simulink model "RuleBasedTractionControl"  (R2019b)
settings: Solver=ode1  StartTime=0.0  StopTime=inf  FixedStep=0.0002  RelTol=1e-3
PreLoadFcn:
  | vehicle = 'Car'; if ~length(which('cmself')), cmenv; end
  | RuleBasedTractionControl_bus
InitFcn:
  | vehicle = 'Car'; if ~length(which('cmself')), cmenv; end
  | RuleBasedTractionControl_bus
model workspace (MAT data in the model file):
  SLIP_FRONT = [0 0.05 0.1 0.15 0.25 0.5 1 2 10]
  TORQUE_DELTA_FRONT = [0 0.03 0.07 0.09 0.15 0.25 0.5 0.8 1]
libraries: CarMaker4SL x4
(part 2 of 2)

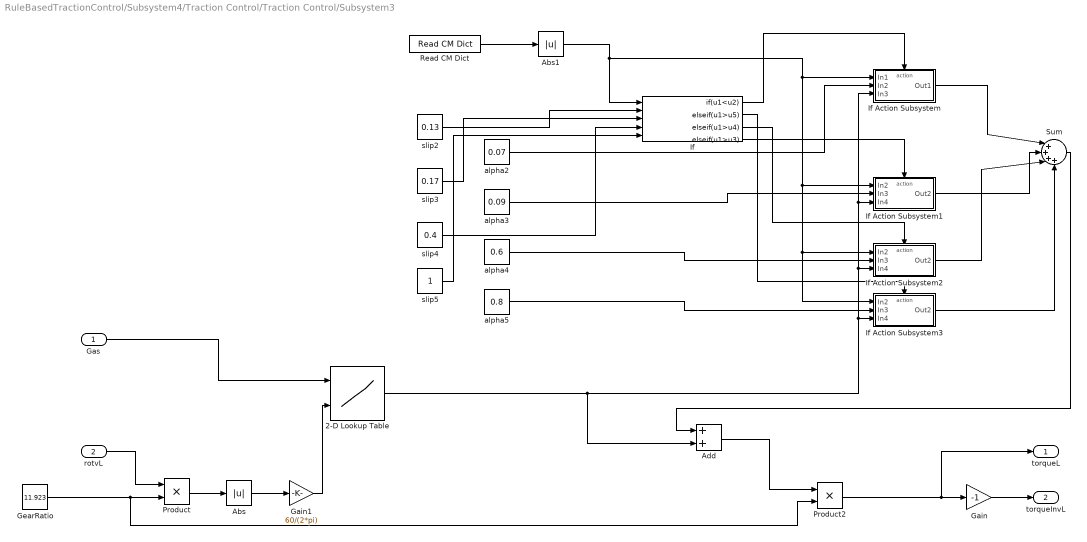
== system RuleBasedTractionControl/Subsystem4/Traction Control/Traction Control/Subsystem3 ==
  Gas : Inport
  rotvL : Inport  Port=2
  2-D Lookup Table : Lookup_n-D  BreakpointsForDimension1=[0 0.2 0.4 0.6 0.8 1]  BreakpointsForDimension2=[0 2000 4000 6000 8000 10000 12000 14000 15000 16000 17000 18000 20000 22000]  Table=[0 0 0 0 0 0 0 0 0 0 0 0 0 0;4 4 4 4 4 4 4 4 4 4 4 4 3 0;8 8 8 8 8 8 8 8 8 8 8 8 6 0;13 13 13 13 13 13 13 13 13 12 12 11 9 0;17 17 17 17 17 17 17 17 17 16 16 15 12 0;21 21 21 21 21 21 21 21 21 20 20 19 15 0]  InternalRulePriority=Speed  RndMeth=Simplest  InputSameDT=on
  Abs : Abs
  Abs1 : Abs
  Add : Sum
  Gain : Gain  Gain=-1
  Gain1 : Gain  Gain=60/(2*pi)
  GearRatio : Constant  Value=11.923
  If : If  NumInputs=5  IfExpression=u1<u2  ElseIfExpressions=u1>u5, u1>u4, u1>u3  ShowElse=off
  If Action Subsystem : Subsystem  TreatAsAtomicUnit=on
  If Action Subsystem1 : Subsystem  TreatAsAtomicUnit=on
  If Action Subsystem2 : Subsystem  TreatAsAtomicUnit=on
  If Action Subsystem3 : Subsystem  TreatAsAtomicUnit=on
  Product : Product
  Product2 : Product
  Read CM Dict : CarMaker4SL/Read CM Dict  xname=Car.LongSlipRR  xsync=off
  Sum : Sum  Inputs=|++++
  alpha2 : Constant  Value=0.07
  alpha3 : Constant  Value=0.09
  alpha4 : Constant  Value=0.6
  alpha5 : Constant  Value=0.8
  slip2 : Constant  Value=0.13
  slip3 : Constant  Value=0.17
  slip4 : Constant  Value=0.4
  slip5 : Constant
  torqueL : Outport
  torqueInvL : Outport  Port=2
  wires:
  Gain/1 -> torqueInvL/1
  Product/1 -> Abs/1
  Gas/1 -> 2-D Lookup Table/1
  GearRatio/1 -> Product2/2, Product/2
  rotvL/1 -> Product/1
  Product2/1 -> Gain/1, torqueL/1
  Abs/1 -> Gain1/1
  Gain1/1 -> 2-D Lookup Table/2
  2-D Lookup Table/1 -> If Action Subsystem3/3(In4), If Action Subsystem2/3(In4), If Action Subsystem1/3(In4), If Action Subsystem/3(In3), Add/2
  Add/1 -> Product2/1
  Read CM Dict/1 -> Abs1/1
  Abs1/1 -> If Action Subsystem3/1(In2), If Action Subsystem2/1(In2), If Action Subsystem1/1(In2), If Action Subsystem/1(In1), If/1
  If/1 -> If Action Subsystem/Action
  If Action Subsystem/1(Out1) -> Sum/1
  If Action Subsystem1/1(Out2) -> Sum/2
  Sum/1 -> Add/1
  alpha2/1 -> If Action Subsystem/2(In2)
  slip2/1 -> If/2
  slip3/1 -> If/3
  slip4/1 -> If/4
  slip5/1 -> If/5
  If/4 -> If Action Subsystem1/Action
  alpha3/1 -> If Action Subsystem1/2(In3)
  If/3 -> If Action Subsystem2/Action
  alpha4/1 -> If Action Subsystem2/2(In3)
  If/2 -> If Action Subsystem3/Action
  alpha5/1 -> If Action Subsystem3/2(In3)
  If Action Subsystem2/1(Out2) -> Sum/3
  If Action Subsystem3/1(Out2) -> Sum/4

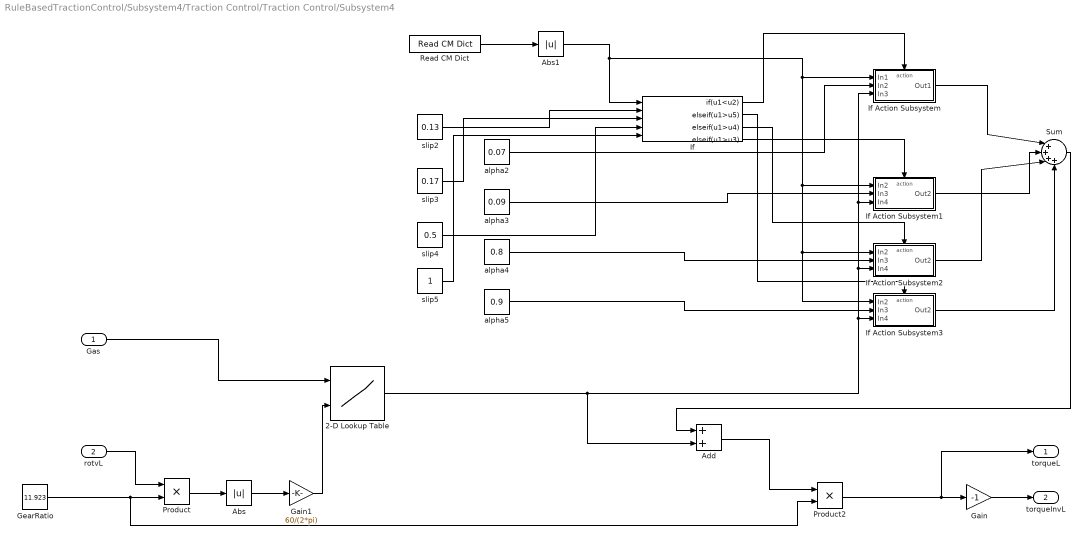
== system RuleBasedTractionControl/Subsystem4/Traction Control/Traction Control/Subsystem4 ==
  Gas : Inport
  rotvL : Inport  Port=2
  2-D Lookup Table : Lookup_n-D  BreakpointsForDimension1=[0 0.2 0.4 0.6 0.8 1]  BreakpointsForDimension2=[0 2000 4000 6000 8000 10000 12000 14000 15000 16000 17000 18000 20000 22000]  Table=[0 0 0 0 0 0 0 0 0 0 0 0 0 0;4 4 4 4 4 4 4 4 4 4 4 4 3 0;8 8 8 8 8 8 8 8 8 8 8 8 6 0;13 13 13 13 13 13 13 13 13 12 12 11 9 0;17 17 17 17 17 17 17 17 17 16 16 15 12 0;21 21 21 21 21 21 21 21 21 20 20 19 15 0]  InternalRulePriority=Speed  RndMeth=Simplest  InputSameDT=on
  Abs : Abs
  Abs1 : Abs
  Add : Sum
  Gain : Gain  Gain=-1
  Gain1 : Gain  Gain=60/(2*pi)
  GearRatio : Constant  Value=11.923
  If : If  NumInputs=5  IfExpression=u1<u2  ElseIfExpressions=u1>u5, u1>u4, u1>u3  ShowElse=off
  If Action Subsystem : Subsystem  TreatAsAtomicUnit=on
  If Action Subsystem1 : Subsystem  TreatAsAtomicUnit=on
  If Action Subsystem2 : Subsystem  TreatAsAtomicUnit=on
  If Action Subsystem3 : Subsystem  TreatAsAtomicUnit=on
  Product : Product
  Product2 : Product
  Read CM Dict : CarMaker4SL/Read CM Dict  xname=Car.LongSlipFL  xsync=off
  Sum : Sum  Inputs=|++++
  alpha2 : Constant  Value=0.07
  alpha3 : Constant  Value=0.09
  alpha4 : Constant  Value=0.8
  alpha5 : Constant  Value=0.9
  slip2 : Constant  Value=0.13
  slip3 : Constant  Value=0.17
  slip4 : Constant  Value=0.5
  slip5 : Constant
  torqueL : Outport
  torqueInvL : Outport  Port=2
  wires:
  Gain/1 -> torqueInvL/1
  Product/1 -> Abs/1
  Gas/1 -> 2-D Lookup Table/1
  GearRatio/1 -> Product2/2, Product/2
  rotvL/1 -> Product/1
  Product2/1 -> Gain/1, torqueL/1
  Abs/1 -> Gain1/1
  Gain1/1 -> 2-D Lookup Table/2
  2-D Lookup Table/1 -> If Action Subsystem3/3(In4), If Action Subsystem2/3(In4), If Action Subsystem1/3(In4), If Action Subsystem/3(In3), Add/2
  Add/1 -> Product2/1
  Read CM Dict/1 -> Abs1/1
  Abs1/1 -> If Action Subsystem3/1(In2), If Action Subsystem2/1(In2), If Action Subsystem1/1(In2), If Action Subsystem/1(In1), If/1
  If/1 -> If Action Subsystem/Action
  If Action Subsystem/1(Out1) -> Sum/1
  If Action Subsystem1/1(Out2) -> Sum/2
  Sum/1 -> Add/1
  alpha2/1 -> If Action Subsystem/2(In2)
  slip2/1 -> If/2
  slip3/1 -> If/3
  slip4/1 -> If/4
  slip5/1 -> If/5
  If/4 -> If Action Subsystem1/Action
  alpha3/1 -> If Action Subsystem1/2(In3)
  If/3 -> If Action Subsystem2/Action
  alpha4/1 -> If Action Subsystem2/2(In3)
  If/2 -> If Action Subsystem3/Action
  alpha5/1 -> If Action Subsystem3/2(In3)
  If Action Subsystem2/1(Out2) -> Sum/3
  If Action Subsystem3/1(Out2) -> Sum/4

== system RuleBasedTractionControl/Subsystem4/Launch Control/LaunchControl/Subsystem/If Action Subsystem ==
  In1 : Inport
  Action Port : ActionPort  ActionPortLabel=if(u2< u1)
  Out1 : Outport
  wires:
  In1/1 -> Out1/1

== system RuleBasedTractionControl/Subsystem4/Launch Control/LaunchControl/Subsystem/If Action Subsystem1 ==
  In1 : Inport
  Action Port : ActionPort  ActionPortLabel=else
  Out1 : Outport
  wires:
  In1/1 -> Out1/1

== system RuleBasedTractionControl/Subsystem4/Launch Control/LaunchControl/Subsystem1/If Action Subsystem ==
  In1 : Inport
  Action Port : ActionPort  ActionPortLabel=if(u2< u1)
  Out1 : Outport
  wires:
  In1/1 -> Out1/1

== system RuleBasedTractionControl/Subsystem4/Launch Control/LaunchControl/Subsystem1/If Action Subsystem1 ==
  In1 : Inport
  Action Port : ActionPort  ActionPortLabel=else
  Out1 : Outport
  wires:
  In1/1 -> Out1/1

== system RuleBasedTractionControl/Subsystem4/Launch Control/LaunchControl/Subsystem2/If Action Subsystem ==
  In1 : Inport
  Action Port : ActionPort  ActionPortLabel=if(u2< u1)
  Out1 : Outport
  wires:
  In1/1 -> Out1/1

== system RuleBasedTractionControl/Subsystem4/Launch Control/LaunchControl/Subsystem2/If Action Subsystem1 ==
  In1 : Inport
  Action Port : ActionPort  ActionPortLabel=else
  Out1 : Outport
  wires:
  In1/1 -> Out1/1

== system RuleBasedTractionControl/Subsystem4/Launch Control/LaunchControl/Subsystem3/If Action Subsystem ==
  In1 : Inport
  Action Port : ActionPort  ActionPortLabel=if(u2< u1)
  Out1 : Outport
  wires:
  In1/1 -> Out1/1

== system RuleBasedTractionControl/Subsystem4/Launch Control/LaunchControl/Subsystem3/If Action Subsystem1 ==
  In1 : Inport
  Action Port : ActionPort  ActionPortLabel=else
  Out1 : Outport
  wires:
  In1/1 -> Out1/1

== system RuleBasedTractionControl/Subsystem4/Traction Control/Traction Control/Subsystem1/If Action Subsystem ==
  In1 : Inport
  In2 : Inport  Port=2
  In3 : Inport  Port=3
  Action Port : ActionPort  ActionPortLabel=if(u1<u2)
  Product : Product  Inputs=3
  Out1 : Outport
  wires:
  In1/1 -> Product/1
  In2/1 -> Product/2
  In3/1 -> Product/3
  Product/1 -> Out1/1

== system RuleBasedTractionControl/Subsystem4/Traction Control/Traction Control/Subsystem1/If Action Subsystem1 ==
  In2 : Inport
  In3 : Inport  Port=2
  In4 : Inport  Port=3
  Action Port : ActionPort  ActionPortLabel=elseif( u1>u3)
  Constant : Constant  Value=-1
  Product : Product  Inputs=4
  Out2 : Outport
  wires:
  In4/1 -> Product/3
  In3/1 -> Product/2
  In2/1 -> Product/1
  Product/1 -> Out2/1
  Constant/1 -> Product/4

== system RuleBasedTractionControl/Subsystem4/Traction Control/Traction Control/Subsystem1/If Action Subsystem2 ==
  In2 : Inport
  In3 : Inport  Port=2
  In4 : Inport  Port=3
  Action Port : ActionPort  ActionPortLabel=elseif( u1>u4)
  Constant : Constant  Value=-1
  Product : Product  Inputs=4
  Out2 : Outport
  wires:
  In4/1 -> Product/3
  In3/1 -> Product/2
  In2/1 -> Product/1
  Product/1 -> Out2/1
  Constant/1 -> Product/4

== system RuleBasedTractionControl/Subsystem4/Traction Control/Traction Control/Subsystem1/If Action Subsystem3 ==
  In2 : Inport
  In3 : Inport  Port=2
  In4 : Inport  Port=3
  Action Port : ActionPort  ActionPortLabel=elseif(u1>u5)
  Constant : Constant  Value=-1
  Product : Product  Inputs=4
  Out2 : Outport
  wires:
  In4/1 -> Product/3
  In3/1 -> Product/2
  In2/1 -> Product/1
  Product/1 -> Out2/1
  Constant/1 -> Product/4

== system RuleBasedTractionControl/Subsystem4/Traction Control/Traction Control/Subsystem2/If Action Subsystem ==
  In1 : Inport
  In2 : Inport  Port=2
  In3 : Inport  Port=3
  Action Port : ActionPort  ActionPortLabel=if(u1<u2)
  Product : Product  Inputs=3
  Out1 : Outport
  wires:
  In1/1 -> Product/1
  In2/1 -> Product/2
  In3/1 -> Product/3
  Product/1 -> Out1/1

== system RuleBasedTractionControl/Subsystem4/Traction Control/Traction Control/Subsystem2/If Action Subsystem1 ==
  In2 : Inport
  In3 : Inport  Port=2
  In4 : Inport  Port=3
  Action Port : ActionPort  ActionPortLabel=elseif( u1>u3)
  Constant : Constant  Value=-1
  Product : Product  Inputs=4
  Out2 : Outport
  wires:
  In4/1 -> Product/3
  In3/1 -> Product/2
  In2/1 -> Product/1
  Product/1 -> Out2/1
  Constant/1 -> Product/4

== system RuleBasedTractionControl/Subsystem4/Traction Control/Traction Control/Subsystem2/If Action Subsystem2 ==
  In2 : Inport
  In3 : Inport  Port=2
  In4 : Inport  Port=3
  Action Port : ActionPort  ActionPortLabel=elseif( u1>u4)
  Constant : Constant  Value=-1
  Product : Product  Inputs=4
  Out2 : Outport
  wires:
  In4/1 -> Product/3
  In3/1 -> Product/2
  In2/1 -> Product/1
  Product/1 -> Out2/1
  Constant/1 -> Product/4

== system RuleBasedTractionControl/Subsystem4/Traction Control/Traction Control/Subsystem2/If Action Subsystem3 ==
  In2 : Inport
  In3 : Inport  Port=2
  In4 : Inport  Port=3
  Action Port : ActionPort  ActionPortLabel=elseif(u1>u5)
  Constant : Constant  Value=-1
  Product : Product  Inputs=4
  Out2 : Outport
  wires:
  In4/1 -> Product/3
  In3/1 -> Product/2
  In2/1 -> Product/1
  Product/1 -> Out2/1
  Constant/1 -> Product/4

== system RuleBasedTractionControl/Subsystem4/Traction Control/Traction Control/Subsystem3/If Action Subsystem ==
  In1 : Inport
  In2 : Inport  Port=2
  In3 : Inport  Port=3
  Action Port : ActionPort  ActionPortLabel=if(u1<u2)
  Product : Product  Inputs=3
  Out1 : Outport
  wires:
  In1/1 -> Product/1
  In2/1 -> Product/2
  In3/1 -> Product/3
  Product/1 -> Out1/1

== system RuleBasedTractionControl/Subsystem4/Traction Control/Traction Control/Subsystem3/If Action Subsystem1 ==
  In2 : Inport
  In3 : Inport  Port=2
  In4 : Inport  Port=3
  Action Port : ActionPort  ActionPortLabel=elseif( u1>u3)
  Constant : Constant  Value=-1
  Product : Product  Inputs=4
  Out2 : Outport
  wires:
  In4/1 -> Product/3
  In3/1 -> Product/2
  In2/1 -> Product/1
  Product/1 -> Out2/1
  Constant/1 -> Product/4

== system RuleBasedTractionControl/Subsystem4/Traction Control/Traction Control/Subsystem3/If Action Subsystem2 ==
  In2 : Inport
  In3 : Inport  Port=2
  In4 : Inport  Port=3
  Action Port : ActionPort  ActionPortLabel=elseif( u1>u4)
  Constant : Constant  Value=-1
  Product : Product  Inputs=4
  Out2 : Outport
  wires:
  In4/1 -> Product/3
  In3/1 -> Product/2
  In2/1 -> Product/1
  Product/1 -> Out2/1
  Constant/1 -> Product/4

== system RuleBasedTractionControl/Subsystem4/Traction Control/Traction Control/Subsystem3/If Action Subsystem3 ==
  In2 : Inport
  In3 : Inport  Port=2
  In4 : Inport  Port=3
  Action Port : ActionPort  ActionPortLabel=elseif(u1>u5)
  Constant : Constant  Value=-1
  Product : Product  Inputs=4
  Out2 : Outport
  wires:
  In4/1 -> Product/3
  In3/1 -> Product/2
  In2/1 -> Product/1
  Product/1 -> Out2/1
  Constant/1 -> Product/4

== system RuleBasedTractionControl/Subsystem4/Traction Control/Traction Control/Subsystem4/If Action Subsystem ==
  In1 : Inport
  In2 : Inport  Port=2
  In3 : Inport  Port=3
  Action Port : ActionPort  ActionPortLabel=if(u1<u2)
  Product : Product  Inputs=3
  Out1 : Outport
  wires:
  In1/1 -> Product/1
  In2/1 -> Product/2
  In3/1 -> Product/3
  Product/1 -> Out1/1

== system RuleBasedTractionControl/Subsystem4/Traction Control/Traction Control/Subsystem4/If Action Subsystem1 ==
  In2 : Inport
  In3 : Inport  Port=2
  In4 : Inport  Port=3
  Action Port : ActionPort  ActionPortLabel=elseif( u1>u3)
  Constant : Constant  Value=-1
  Product : Product  Inputs=4
  Out2 : Outport
  wires:
  In4/1 -> Product/3
  In3/1 -> Product/2
  In2/1 -> Product/1
  Product/1 -> Out2/1
  Constant/1 -> Product/4

== system RuleBasedTractionControl/Subsystem4/Traction Control/Traction Control/Subsystem4/If Action Subsystem2 ==
  In2 : Inport
  In3 : Inport  Port=2
  In4 : Inport  Port=3
  Action Port : ActionPort  ActionPortLabel=elseif( u1>u4)
  Constant : Constant  Value=-1
  Product : Product  Inputs=4
  Out2 : Outport
  wires:
  In4/1 -> Product/3
  In3/1 -> Product/2
  In2/1 -> Product/1
  Product/1 -> Out2/1
  Constant/1 -> Product/4

== system RuleBasedTractionControl/Subsystem4/Traction Control/Traction Control/Subsystem4/If Action Subsystem3 ==
  In2 : Inport
  In3 : Inport  Port=2
  In4 : Inport  Port=3
  Action Port : ActionPort  ActionPortLabel=elseif(u1>u5)
  Constant : Constant  Value=-1
  Product : Product  Inputs=4
  Out2 : Outport
  wires:
  In4/1 -> Product/3
  In3/1 -> Product/2
  In2/1 -> Product/1
  Product/1 -> Out2/1
  Constant/1 -> Product/4
